simulink model "sim_polytrajD3"  (R2020b)
settings: Solver=VariableStepAuto  StartTime=0.0  StopTime=10.0  RelTol=1e-3
libraries: simulink x1
settings Model: Creator=mstra  LastModifiedBy=mstra

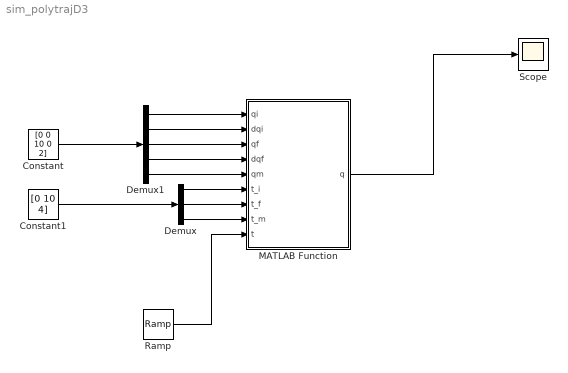
== system sim_polytrajD3 ==
  Constant : Constant  Value=[0 0 10 0 2]
  Constant1 : Constant  Value=[0 10 4]
  Demux : Demux  Outputs=3
  Demux1 : Demux  Outputs=5
  MATLAB Function : MATLAB Function  TreatAsAtomicUnit=on
  Ramp : simulink/Sources/Ramp  slope=1  start=0  InitialOutput=0
  Scope : Scope
  wires:
  Demux/1 -> MATLAB Function/6(t_i)
  Demux/2 -> MATLAB Function/7(t_f)
  Demux1/1 -> MATLAB Function/1(qi)
  Demux1/4 -> MATLAB Function/4(dqf)
  Constant1/1 -> Demux/1
  Constant/1 -> Demux1/1
  Ramp/1 -> MATLAB Function/9(t)
  MATLAB Function/1(q) -> Scope/1
  Demux1/2 -> MATLAB Function/2(dqi)
  Demux1/3 -> MATLAB Function/3(qf)
  Demux1/5 -> MATLAB Function/5(qm)
  Demux/3 -> MATLAB Function/8(t_m)

== matlab function sim_polytrajD3/MATLAB Function ==
  data: qi input; dqi input; q output; qf input; dqf input; qm input; t_i input; t_f input; t_m input; t input
function q  = poly_trajD3(qi, dqi, qf, dqf, qm, t_i, t_f, t_m, t)
%makes polynomial from inputs

%makes polynomial from inputs

v = [qi dqi qf dqf qm]';

A = [1 t_i t_i^2 t_i^3 t_i^4;
    0 1 2*t_i 3*t_i^2 4*t_i^3;
    1 t_f t_f^2 t_f^3 t_f^4;
    0 1 2*t_f 3*t_f^2 4*t_f^3;
    1 t_m t_m^2 t_m^3 t_m^4];

% invert to get the coefficients
a = inv(A)*v;
% trying the matrix way
q = qi + dqi.*(t-t_i) + a(3,1).*(t-t_i)^2 + a(4,1).*(t-t_i)^3 + a(5,1).*(t-t_i)^4;
% return posit_ion at t
end
